simulink model "dspcvsd"  (Simulink 5.0)
settings: Solver=ode5  SolverMode=SingleTasking  StartTime=0.0  StopTime=99999  FixedStep=1/64000  MaxStep=1/64000  RelTol=1e-3  AbsTol=1e-6
values from neighbouring files (symbols this model uses):
  D = var(Noisef)    [lmsxy.m]
libraries: dspwvfmcdlib x3, simulink3 x2, dsparch3 x1, dspsigattribs x1, dspbuff3 x1, dspsigops x1
settings Model: RequirementInfo=9  Creator=don  LastModifiedBy=mkhan  ExtModeTrigMode=oneshot  ExtModeArmWhenConnect=off  SaveTime=off  SaveOutput=off  LimitDataPoints=off  SignalLoggingName=logsOut  IntegerOverflowMsg=none  BlockReductionOpt=off  BooleanDataType=off  ZeroCrossControl=UseLocalSettings  TargetHWChar=2  TargetHWWordLengths=8,16,32,32  RTWMathFcnLibMatFile=iso_c_tmw.mat  RTWOptions="-aEnforceIntegerDowncast=1 -aFoldNonRolledExpr=1 -aInlineInvariantSignals=1 -aInlineParameters=0 -aLocalBlockOutputs=1 -aRollThreshold=5 -aRTWVerbose=1 -aForceParamTrailComments=0 -aGenerateComments=1 -aIgnoreCustomStorageClasses=1 -aIncHierarchyInIds=0 -aMaxRTWIdLen=31 -aShowEliminatedStatements=0 -aReadOnly=0 -aTargetFcnLib=\"iso_c_tmw.mat\" -aIncDataTypeInIds=0 -aPrefixModelToSubsysFcnNames=1 -aInlinedPrmAccess=\"Literals\" -aGenerateFullHeader=1 -aIsPILTarget=0 -aGenerateReport=0 -aLogVarNameModifier=\"rt_\" -aExtMode=0 -aExtModeStaticAlloc=0 -aExtModeTesting=0 -aExtModeStaticAllocSize=1000000 -aExtModeTransport=0"

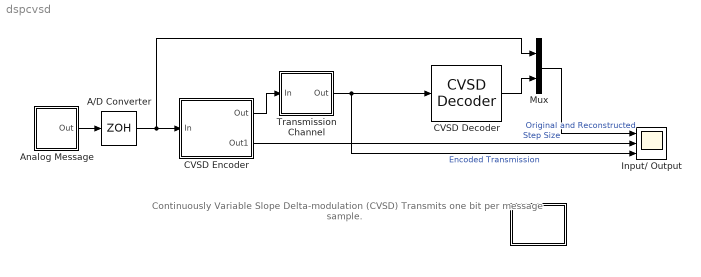
== system dspcvsd ==
  note: Continuously Variable Slope
      | Delta-modulation (CVSD)
      |
      | Transmits one bit per message sample.
  " " : Subsystem
      mask Type: CVSD Demo Info
      mask Display: disp('Info')
  A/D Converter : ZeroOrderHold  SampleTime=1/8000
  Analog Message : Subsystem
  CVSD Decoder : dspwvfmcdlib/CVSD Decoder  DeltaMax=20  SylIntTau=0.99  DeltaMin=0.01  RecIntTau=0.96
  CVSD Encoder : Subsystem  AncestorBlock=dspwvfmcdlib/CVSD Encoder  mask(CVSD Encoder){EncDeltaMax=20, EncSylIntTau=0.99, EncDeltaMin=0.01, EncRecIntTau=0.96}
      mask prompts: EncDeltaMax "Maximum step size"; EncSylIntTau "Syllabic integrator time constant"; EncDeltaMin "Minimum step size"; EncRecIntTau "Reconstruction integrator time constant"
      mask Display: disp('CVSD\nEncoder')
  Input/ Output : Scope  NumInputPorts=3
      settings: TimeRange=0.02  YMin=-2~-5~-0.1  YMax=2~5~1.1  DataFormat=Array
  Mux : Mux  Inputs=2
  Transmission Channel : Subsystem
  wires:
  Mux/1 -> Input/ Output/1  "Original and Reconstructed"
  Transmission Channel/1(Out) -> CVSD Decoder/1, Input/ Output/3  "Encoded Transmission"
  Analog Message/1(Out) -> A/D Converter/1
  CVSD Decoder/1 -> Mux/2
  CVSD Encoder/1(Out) -> Transmission Channel/1(In)
  CVSD Encoder/2(Out1) -> Input/ Output/2  "Step Size"
  A/D Converter/1 -> CVSD Encoder/1(In), Mux/1

== system dspcvsd/  ==
  note: Continuously Variable Slope Delta-Modulation (CVSD) is a modification of Delta Modulation.
      |
      | Delta-Modulation (DM) is a differential waveform quantization (or coding) technique. A DM
      | encoder uses the error between the original signal to be coded and the coded signal itself to
      | create a differentially-quantized data stream. This data stream (usually the computer error
      | signal) is a lower-bit-rate signal that can be decoded by a matched decoder on the receiver
      | side in order to achieve data compression and hence low data transmission rates.
      |
      | CVSD has an adaptive step-size. In the encoded bit-stream, each "1" bit means "increase the
      | amplitude" by the step-size (as compared to the previous decoded signal sample), while a
      |  "0" bit means "decrease the amplitude"  by the step-size (as compared to the previous
      | decoded signal sample. By adjusting (adapting) the step-size to the changes in slope of the
      | input signal, the encoder is able to represent low-frequency signals with greater accuracy
      | without sacrificing as much performance due to "slope-overload" at higher frequencies. When
      |  the slope of the input signal changes too quickly for the encoder to keep up with it, the
      | step-size is increased. Conversely, when the input signal slope changes slowly, the step-size
      | is decreased. A slope-overload detector and syllabic filter is used in conjunction with a pulse
      | amplitude modulator (PAM) to accomplish the step-size adaption.

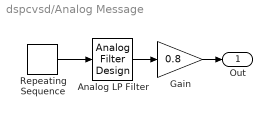
== system dspcvsd/Analog Message ==
  Analog LP Filter : dsparch3/Analog Filter Design  method=Butterworth  filttype=Lowpass  N=5  Wlo=2*pi*400  Whi=80  Rp=3  Rs=40
  Gain : Gain  Gain=0.8  SaturateOnIntegerOverflow=on
  Repeating Sequence : simulink3/Sources/Repeating Sequence  rep_seq_t=[0 .005 .005 .015 .015 .02]  rep_seq_y=[1 1 -1 -1 1 1]
  Out : Outport  InitialOutput=0
  wires:
  Analog LP Filter/1 -> Gain/1
  Repeating Sequence/1 -> Analog LP Filter/1
  Gain/1 -> Out/1

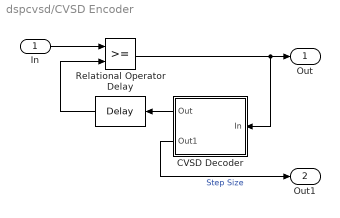
== system dspcvsd/CVSD Encoder ==
  In : Inport
  CVSD Decoder : Subsystem  Orientation=left  AncestorBlock=dspwvfmcdlib/CVSD Decoder  mask(CVSD Decoder){DeltaMax=EncDeltaMax, SylIntTau=EncSylIntTau, DeltaMin=EncDeltaMin, RecIntTau=EncRecIntTau}
      mask prompts: DeltaMax "Maximum step size"; SylIntTau "Syllabic integrator time constant"; DeltaMin "Minimum step size"; RecIntTau "Reconstruction integrator time constant"
      mask Display: disp('CVSD\nDecoder')
  Delay : dspsigops/Delay  Orientation=left  dly_unit=Samples  delay=1  ic_detail=on  dif_ic_for_ch=off  dif_ic_for_dly=off  ic=0  reset_popup=None
  Relational Operator : RelationalOperator  InputSameDT=on
  Out : Outport
  Out1 : Outport  Port=2
  wires:
  Relational Operator/1 -> CVSD Decoder/1(In), Out/1
  In/1 -> Relational Operator/1
  Delay/1 -> Relational Operator/2
  CVSD Decoder/1(Out) -> Delay/1
  CVSD Decoder/2(Out1) -> Out1/1  "Step Size"

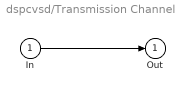
== system dspcvsd/Transmission Channel ==
  In : Inport
  Out : Outport  InitialOutput=0
  wires:
  In/1 -> Out/1

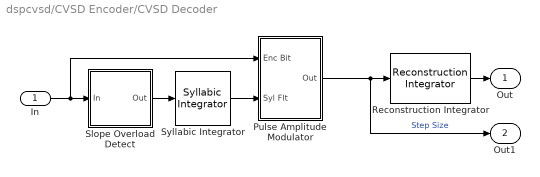
== system dspcvsd/CVSD Encoder/CVSD Decoder ==
  In : Inport
  Pulse Amplitude Modulator : Subsystem
  Reconstruction Integrator : dspwvfmcdlib/CVSD Decoder/Reconstruction Integrator
  Slope Overload Detect : Subsystem
      mask Display: disp('Slope\nOverload\nDetect')
  Syllabic Integrator : dspwvfmcdlib/CVSD Decoder/Syllabic Integrator
  Out : Outport
  Out1 : Outport  Port=2
  wires:
  In/1 -> Slope Overload Detect/1(In), Pulse Amplitude Modulator/1(Enc Bit)
  Pulse Amplitude Modulator/1(Out) -> Reconstruction Integrator/1, Out1/1  "Step Size"
  Reconstruction Integrator/1 -> Out/1
  Slope Overload Detect/1(Out) -> Syllabic Integrator/1
  Syllabic Integrator/1 -> Pulse Amplitude Modulator/2(Syl Flt)

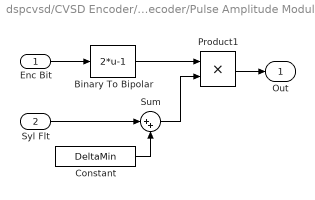
== system dspcvsd/CVSD Encoder/CVSD Decoder/Pulse Amplitude Modulator ==
  Enc Bit : Inport
  Syl Flt : Inport  Port=2
  Binary To Bipolar : Fcn  Expr=2*u-1
  Constant : Constant  Value=DeltaMin
  Product1 : Product  SaturateOnIntegerOverflow=on  RndMeth=Zero  InputSameDT=on
  Sum : Sum  Inputs=|++  SaturateOnIntegerOverflow=on  InputSameDT=on
  Out : Outport
  wires:
  Product1/1 -> Out/1
  Constant/1 -> Sum/2
  Syl Flt/1 -> Sum/1
  Sum/1 -> Product1/2
  Binary To Bipolar/1 -> Product1/1
  Enc Bit/1 -> Binary To Bipolar/1

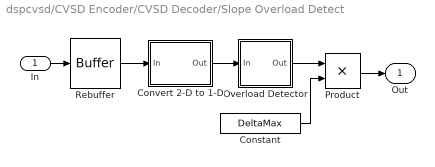
== system dspcvsd/CVSD Encoder/CVSD Decoder/Slope Overload Detect ==
  In : Inport
  Constant : Constant  Value=DeltaMax
  Convert 2-D to 1-D : Subsystem  AncestorBlock=dspelem3/Convert 2-D to 1-D
      mask Type: Convert 2-D to 1-D
      mask Description: Output a (1-D) vector signal.
      mask Display: disp('U( : )')
  Overload Detector : Subsystem
      mask Display: disp('Overload\nDetector')
  Product : Product  SaturateOnIntegerOverflow=on  RndMeth=Zero  InputSameDT=on
  Rebuffer : dspbuff3/Buffer  N=3  V=2  ic=0
  Out : Outport
  wires:
  Product/1 -> Out/1
  In/1 -> Rebuffer/1
  Constant/1 -> Product/2
  Overload Detector/1(Out) -> Product/1
  Convert 2-D to 1-D/1(Out) -> Overload Detector/1(In)
  Rebuffer/1 -> Convert 2-D to 1-D/1(In)

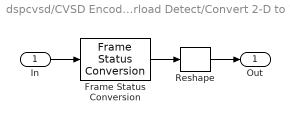
== system dspcvsd/CVSD Encoder/CVSD Decoder/Slope Overload Detect/Convert 2-D to 1-D ==
  In : Inport
  Frame Status Conversion : dspsigattribs/Frame Status Conversion  growRefPort=off  outframe=Sample-based
  Reshape : simulink3/Signals & Systems/Reshape  OutputDimensionality=1-D array  OutputDimensions=[1,1]
  Out : Outport
  wires:
  Frame Status Conversion/1 -> Reshape/1
  In/1 -> Frame Status Conversion/1
  Reshape/1 -> Out/1

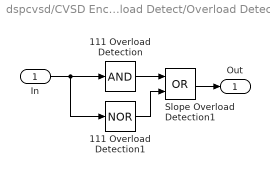
== system dspcvsd/CVSD Encoder/CVSD Decoder/Slope Overload Detect/Overload Detector ==
  In : Inport
  111 Overload Detection : Logic  Inputs=1
  111 Overload Detection1 : Logic  Operator=NOR  Inputs=1
  Slope Overload Detection1 : Logic  Operator=OR
  Out : Outport
  wires:
  111 Overload Detection/1 -> Slope Overload Detection1/1
  111 Overload Detection1/1 -> Slope Overload Detection1/2
  In/1 -> 111 Overload Detection/1, 111 Overload Detection1/1
  Slope Overload Detection1/1 -> Out/1
